simulink model "eovsa_corr_300mhz"  (R2012b)
(part 2 of 65)

      | % elseif strcmp(mode, 'fields of arbitrary size')
      | %     current_names = textscan(strtrim(strrep(strrep(get_param(blk, 'names'), ']', ''), '[', '')), '%s');
      | %     current_names = current_names{1};
      | %     numios = length(current_names);
      | %     if length(current_bins) ~= numios,
      | %         error('%d field names specified, but %d binary pts?', numios, length(current_bins));
      | %     end
      | % end
  vector_acc : Subsystem  mask{fpga_clk=300, fft_size=12, n_pps=50}
      mask prompts: fpga_clk "FPGA Clock Frequency (MHz)"; fft_size "FFT channels (2 ^ ?)"; n_pps "Accumulatioms per second"
  x_dv_count0 : Subsystem  Tag=xps:sw_reg  AncestorBlock=xps_library/software_register  mask(swreg){mode=one value, io_dir=To Processor, io_delay=0, sample_period=1, names=reg, bitwidths=32, arith_types=0, bin_pts=0, sim_port=on, show_format=off}
      mask prompts: io_dir "I/O direction"; io_delay "I/O delay"; sample_period "Sample period"; names "Name:"; bitwidths "Bitwidth:"; arith_types "Type (ufix=0, fix=1, bool=2):"; bin_pts "Binary pt:"; sim_port "Provide sim input/output?"; show_format "Print format string?"
      mask init:
      | swreg_init(gcb)
      settings: AttributesFormatString=1output
      mask TypeOptions mode: one value | fields of equal size | fields of arbitrary size
      mask Callback mode: swreg_cb(gcb);
      mask TypeOptions io_dir: To Processor | From Processor
      mask Callback io_dir:
      | mask_enables = get_param(gcb, 'MaskEnables');
      | mask_names = get_param(gcb, 'MaskNames');
      | if strcmp(get_param(gcb, 'io_dir'), 'To Processor'),
      |     mask_enables{ismember(mask_names, 'sample_period')} = 'off';
      | else
      |     mask_enables{ismember(mask_names, 'sample_period')} = 'on';
      | end
      | set_param(gcb, 'MaskEnables', mask_enables);
      mask Callback bitwidths:
      | swreg_maskcheck(gcb);
      | % blk = gcb;
      | % mode = get_param(blk, 'mode');
      | % current_widths = eval(get_param(blk, 'bitwidths'));
      | % if (strcmp(mode, 'one value') || strcmp(mode, 'fields of equal size')) && (length(current_widths) > 1),
      | %     error('Only one width may be specified for this mode.');
      | % elseif strcmp(mode, 'fields of arbitrary size')
      | %     current_names = textscan(strtrim(strrep(strrep(get_param(blk, 'names'), ']', ''), '[', '')), '%s');
      | %     current_names = current_names{1};
      | %     numios = length(current_names);
      | %     if length(current_widths) ~= numios,
      | %         error('%d field names specified, but %d widths?', numios, length(current_widths));
      | %     end
      | % end
      | % total_width = 0;
      | % for ctr = 1 : length(current_widths),
      | %     total_width = total_width + current_widths(ctr);
      | % end
      | % if total_width > 32,
      | %     error('Total width must be 32 or less, set to %d.', total_width);
      | % end
      mask Callback arith_types:
      | [numios, ~, ~, ~, current_types] = swreg_maskcheck(gcb);
      | % blk = gcb;
      | % mode = get_param(blk, 'mode');
      | % current_types = eval(get_param(blk, 'arith_types'));
      | % numios = length(current_types);
      | % if (strcmp(mode, 'one value') || strcmp(mode, 'fields of equal size')) && (length(current_types) > 1),
      | %     error('Only one type may be specified for this mode.');
      | % elseif strcmp(mode, 'fields of arbitrary size')
      | %     current_names = textscan(strtrim(strrep(strrep(get_param(blk, 'names'), ']', ''), '[', '')), '%s');
      | %     current_names = current_names{1};
      | %     numios = length(current_names);
      | %     if length(current_types) ~= numios,
      | %         error('%d field names specified, but %d types?', numios, length(current_types));
      | %     end
      | % end
      | problem = 0;
      | for ctr = 1 : numios,
      |     t = current_types(ctr);
      |     if (t < 0) || (t > 2),
      |         problem = t;
      |         ctr = numios + 1;
      |     end
      | end
      | if problem ~= 0,
      |     error('Type cannot be %i, must be 0, 1 or 2.', problem);
      | end
      mask Callback bin_pts:
      | swreg_maskcheck(gcb);
      | % blk = gcb;
      | % mode = get_param(blk, 'mode');
      | % current_bins = eval(get_param(blk, 'bin_pts'));
      | % if (strcmp(mode, 'one value') || strcmp(mode, 'fields of equal size')) && (length(current_bins) > 1),
      | %     error('Only one binary pt may be specified for this mode.');
      | % elseif strcmp(mode, 'fields of arbitrary size')
      | %     current_names = textscan(strtrim(strrep(strrep(get_param(blk, 'names'), ']', ''), '[', '')), '%s');
      | %     current_names = current_names{1};
      | %     numios = length(current_names);
      | %     if length(current_bins) ~= numios,
      | %         error('%d field names specified, but %d binary pts?', numios, length(current_bins));
      | %     end
      | % end
  x_dv_count1 : Subsystem  Tag=xps:sw_reg  AncestorBlock=xps_library/software_register  mask(swreg){mode=one value, io_dir=To Processor, io_delay=0, sample_period=1, names=reg, bitwidths=32, arith_types=0, bin_pts=0, sim_port=on, show_format=off}
      mask prompts: io_dir "I/O direction"; io_delay "I/O delay"; sample_period "Sample period"; names "Name:"; bitwidths "Bitwidth:"; arith_types "Type (ufix=0, fix=1, bool=2):"; bin_pts "Binary pt:"; sim_port "Provide sim input/output?"; show_format "Print format string?"
      mask init:
      | swreg_init(gcb)
      settings: AttributesFormatString=1output
      mask TypeOptions mode: one value | fields of equal size | fields of arbitrary size
      mask Callback mode: swreg_cb(gcb);
      mask TypeOptions io_dir: To Processor | From Processor
      mask Callback io_dir:
      | mask_enables = get_param(gcb, 'MaskEnables');
      | mask_names = get_param(gcb, 'MaskNames');
      | if strcmp(get_param(gcb, 'io_dir'), 'To Processor'),
      |     mask_enables{ismember(mask_names, 'sample_period')} = 'off';
      | else
      |     mask_enables{ismember(mask_names, 'sample_period')} = 'on';
      | end
      | set_param(gcb, 'MaskEnables', mask_enables);
      mask Callback bitwidths:
      | swreg_maskcheck(gcb);
      | % blk = gcb;
      | % mode = get_param(blk, 'mode');
      | % current_widths = eval(get_param(blk, 'bitwidths'));
      | % if (strcmp(mode, 'one value') || strcmp(mode, 'fields of equal size')) && (length(current_widths) > 1),
      | %     error('Only one width may be specified for this mode.');
      | % elseif strcmp(mode, 'fields of arbitrary size')
      | %     current_names = textscan(strtrim(strrep(strrep(get_param(blk, 'names'), ']', ''), '[', '')), '%s');
      | %     current_names = current_names{1};
      | %     numios = length(current_names);
      | %     if length(current_widths) ~= numios,
      | %         error('%d field names specified, but %d widths?', numios, length(current_widths));
      | %     end
      | % end
      | % total_width = 0;
      | % for ctr = 1 : length(current_widths),
      | %     total_width = total_width + current_widths(ctr);
      | % end
      | % if total_width > 32,
      | %     error('Total width must be 32 or less, set to %d.', total_width);
      | % end
      mask Callback arith_types:
      | [numios, ~, ~, ~, current_types] = swreg_maskcheck(gcb);
      | % blk = gcb;
      | % mode = get_param(blk, 'mode');
      | % current_types = eval(get_param(blk, 'arith_types'));
      | % numios = length(current_types);
      | % if (strcmp(mode, 'one value') || strcmp(mode, 'fields of equal size')) && (length(current_types) > 1),
      | %     error('Only one type may be specified for this mode.');
      | % elseif strcmp(mode, 'fields of arbitrary size')
      | %     current_names = textscan(strtrim(strrep(strrep(get_param(blk, 'names'), ']', ''), '[', '')), '%s');
      | %     current_names = current_names{1};
      | %     numios = length(current_names);
      | %     if length(current_types) ~= numios,
      | %         error('%d field names specified, but %d types?', numios, length(current_types));
      | %     end
      | % end
      | problem = 0;
      | for ctr = 1 : numios,
      |     t = current_types(ctr);
      |     if (t < 0) || (t > 2),
      |         problem = t;
      |         ctr = numios + 1;
      |     end
      | end
      | if problem ~= 0,
      |     error('Type cannot be %i, must be 0, 1 or 2.', problem);
      | end
      mask Callback bin_pts:
      | swreg_maskcheck(gcb);
      | % blk = gcb;
      | % mode = get_param(blk, 'mode');
      | % current_bins = eval(get_param(blk, 'bin_pts'));
      | % if (strcmp(mode, 'one value') || strcmp(mode, 'fields of equal size')) && (length(current_bins) > 1),
      | %     error('Only one binary pt may be specified for this mode.');
      | % elseif strcmp(mode, 'fields of arbitrary size')
      | %     current_names = textscan(strtrim(strrep(strrep(get_param(blk, 'names'), ']', ''), '[', '')), '%s');
      | %     current_names = current_names{1};
      | %     numios = length(current_names);
      | %     if length(current_bins) ~= numios,
      | %         error('%d field names specified, but %d binary pts?', numios, length(current_bins));
      | %     end
      | % end
  x_in_sync_count : Subsystem  Tag=xps:sw_reg  AncestorBlock=xps_library/software_register  mask(swreg){mode=one value, io_dir=To Processor, io_delay=0, sample_period=1, names=reg, bitwidths=32, arith_types=0, bin_pts=0, sim_port=on, show_format=off}
      mask prompts: io_dir "I/O direction"; io_delay "I/O delay"; sample_period "Sample period"; names "Name:"; bitwidths "Bitwidth:"; arith_types "Type (ufix=0, fix=1, bool=2):"; bin_pts "Binary pt:"; sim_port "Provide sim input/output?"; show_format "Print format string?"
      mask init:
      | swreg_init(gcb)
      settings: AttributesFormatString=1output
      mask TypeOptions mode: one value | fields of equal size | fields of arbitrary size
      mask Callback mode: swreg_cb(gcb);
      mask TypeOptions io_dir: To Processor | From Processor
      mask Callback io_dir:
      | mask_enables = get_param(gcb, 'MaskEnables');
      | mask_names = get_param(gcb, 'MaskNames');
      | if strcmp(get_param(gcb, 'io_dir'), 'To Processor'),
      |     mask_enables{ismember(mask_names, 'sample_period')} = 'off';
      | else
      |     mask_enables{ismember(mask_names, 'sample_period')} = 'on';
      | end
      | set_param(gcb, 'MaskEnables', mask_enables);
      mask Callback bitwidths:
      | swreg_maskcheck(gcb);
      | % blk = gcb;
      | % mode = get_param(blk, 'mode');
      | % current_widths = eval(get_param(blk, 'bitwidths'));
      | % if (strcmp(mode, 'one value') || strcmp(mode, 'fields of equal size')) && (length(current_widths) > 1),
      | %     error('Only one width may be specified for this mode.');
      | % elseif strcmp(mode, 'fields of arbitrary size')
      | %     current_names = textscan(strtrim(strrep(strrep(get_param(blk, 'names'), ']', ''), '[', '')), '%s');
      | %     current_names = current_names{1};
      | %     numios = length(current_names);
      | %     if length(current_widths) ~= numios,
      | %         error('%d field names specified, but %d widths?', numios, length(current_widths));
      | %     end
      | % end
      | % total_width = 0;
      | % for ctr = 1 : length(current_widths),
      | %     total_width = total_width + current_widths(ctr);
      | % end
      | % if total_width > 32,
      | %     error('Total width must be 32 or less, set to %d.', total_width);
      | % end
      mask Callback arith_types:
      | [numios, ~, ~, ~, current_types] = swreg_maskcheck(gcb);
      | % blk = gcb;
      | % mode = get_param(blk, 'mode');
      | % current_types = eval(get_param(blk, 'arith_types'));
      | % numios = length(current_types);
      | % if (strcmp(mode, 'one value') || strcmp(mode, 'fields of equal size')) && (length(current_types) > 1),
      | %     error('Only one type may be specified for this mode.');
      | % elseif strcmp(mode, 'fields of arbitrary size')
      | %     current_names = textscan(strtrim(strrep(strrep(get_param(blk, 'names'), ']', ''), '[', '')), '%s');
      | %     current_names = current_names{1};
      | %     numios = length(current_names);
      | %     if length(current_types) ~= numios,
      | %         error('%d field names specified, but %d types?', numios, length(current_types));
      | %     end
      | % end
      | problem = 0;
      | for ctr = 1 : numios,
      |     t = current_types(ctr);
      |     if (t < 0) || (t > 2),
      |         problem = t;
      |         ctr = numios + 1;
      |     end
      | end
      | if problem ~= 0,
      |     error('Type cannot be %i, must be 0, 1 or 2.', problem);
      | end
      mask Callback bin_pts:
      | swreg_maskcheck(gcb);
      | % blk = gcb;
      | % mode = get_param(blk, 'mode');
      | % current_bins = eval(get_param(blk, 'bin_pts'));
      | % if (strcmp(mode, 'one value') || strcmp(mode, 'fields of equal size')) && (length(current_bins) > 1),
      | %     error('Only one binary pt may be specified for this mode.');
      | % elseif strcmp(mode, 'fields of arbitrary size')
      | %     current_names = textscan(strtrim(strrep(strrep(get_param(blk, 'names'), ']', ''), '[', '')), '%s');
      | %     current_names = current_names{1};
      | %     numios = length(current_names);
      | %     if length(current_bins) ~= numios,
      | %         error('%d field names specified, but %d binary pts?', numios, length(current_bins));
      | %     end
      | % end
  x_out_count : Subsystem  Tag=xps:sw_reg  AncestorBlock=xps_library/software_register  mask(swreg){mode=one value, io_dir=To Processor, io_delay=0, sample_period=1, names=reg, bitwidths=32, arith_types=0, bin_pts=0, sim_port=on, show_format=off}
      mask prompts: io_dir "I/O direction"; io_delay "I/O delay"; sample_period "Sample period"; names "Name:"; bitwidths "Bitwidth:"; arith_types "Type (ufix=0, fix=1, bool=2):"; bin_pts "Binary pt:"; sim_port "Provide sim input/output?"; show_format "Print format string?"
      mask init:
      | swreg_init(gcb)
      settings: AttributesFormatString=1output
      mask TypeOptions mode: one value | fields of equal size | fields of arbitrary size
      mask Callback mode: swreg_cb(gcb);
      mask TypeOptions io_dir: To Processor | From Processor
      mask Callback io_dir:
      | mask_enables = get_param(gcb, 'MaskEnables');
      | mask_names = get_param(gcb, 'MaskNames');
      | if strcmp(get_param(gcb, 'io_dir'), 'To Processor'),
      |     mask_enables{ismember(mask_names, 'sample_period')} = 'off';
      | else
      |     mask_enables{ismember(mask_names, 'sample_period')} = 'on';
      | end
      | set_param(gcb, 'MaskEnables', mask_enables);
      mask Callback bitwidths:
      | swreg_maskcheck(gcb);
      | % blk = gcb;
      | % mode = get_param(blk, 'mode');
      | % current_widths = eval(get_param(blk, 'bitwidths'));
      | % if (strcmp(mode, 'one value') || strcmp(mode, 'fields of equal size')) && (length(current_widths) > 1),
      | %     error('Only one width may be specified for this mode.');
      | % elseif strcmp(mode, 'fields of arbitrary size')
      | %     current_names = textscan(strtrim(strrep(strrep(get_param(blk, 'names'), ']', ''), '[', '')), '%s');
      | %     current_names = current_names{1};
      | %     numios = length(current_names);
      | %     if length(current_widths) ~= numios,
      | %         error('%d field names specified, but %d widths?', numios, length(current_widths));
      | %     end
      | % end
      | % total_width = 0;
      | % for ctr = 1 : length(current_widths),
      | %     total_width = total_width + current_widths(ctr);
      | % end
      | % if total_width > 32,
      | %     error('Total width must be 32 or less, set to %d.', total_width);
      | % end
      mask Callback arith_types:
      | [numios, ~, ~, ~, current_types] = swreg_maskcheck(gcb);
      | % blk = gcb;
      | % mode = get_param(blk, 'mode');
      | % current_types = eval(get_param(blk, 'arith_types'));
      | % numios = length(current_types);
      | % if (strcmp(mode, 'one value') || strcmp(mode, 'fields of equal size')) && (length(current_types) > 1),
      | %     error('Only one type may be specified for this mode.');
      | % elseif strcmp(mode, 'fields of arbitrary size')
      | %     current_names = textscan(strtrim(strrep(strrep(get_param(blk, 'names'), ']', ''), '[', '')), '%s');
      | %     current_names = current_names{1};
      | %     numios = length(current_names);
      | %     if length(current_types) ~= numios,
      | %         error('%d field names specified, but %d types?', numios, length(current_types));
      | %     end
      | % end
      | problem = 0;
      | for ctr = 1 : numios,
      |     t = current_types(ctr);
      |     if (t < 0) || (t > 2),
      |         problem = t;
      |         ctr = numios + 1;
      |     end
      | end
      | if problem ~= 0,
      |     error('Type cannot be %i, must be 0, 1 or 2.', problem);
      | end
      mask Callback bin_pts:
      | swreg_maskcheck(gcb);
      | % blk = gcb;
      | % mode = get_param(blk, 'mode');
      | % current_bins = eval(get_param(blk, 'bin_pts'));
      | % if (strcmp(mode, 'one value') || strcmp(mode, 'fields of equal size')) && (length(current_bins) > 1),
      | %     error('Only one binary pt may be specified for this mode.');
      | % elseif strcmp(mode, 'fields of arbitrary size')
      | %     current_names = textscan(strtrim(strrep(strrep(get_param(blk, 'names'), ']', ''), '[', '')), '%s');
      | %     current_names = current_names{1};
      | %     numios = length(current_names);
      | %     if length(current_bins) ~= numios,
      | %         error('%d field names specified, but %d binary pts?', numios, length(current_bins));
      | %     end
      | % end
  x_packet_count : Subsystem  Tag=xps:sw_reg  AncestorBlock=xps_library/software_register  mask(swreg){mode=one value, io_dir=To Processor, io_delay=0, sample_period=1, names=reg, bitwidths=32, arith_types=0, bin_pts=0, sim_port=on, show_format=off}
      mask prompts: io_dir "I/O direction"; io_delay "I/O delay"; sample_period "Sample period"; names "Name:"; bitwidths "Bitwidth:"; arith_types "Type (ufix=0, fix=1, bool=2):"; bin_pts "Binary pt:"; sim_port "Provide sim input/output?"; show_format "Print format string?"
      mask init:
      | swreg_init(gcb)
      settings: AttributesFormatString=1output
      mask TypeOptions mode: one value | fields of equal size | fields of arbitrary size
      mask Callback mode: swreg_cb(gcb);
      mask TypeOptions io_dir: To Processor | From Processor
      mask Callback io_dir:
      | mask_enables = get_param(gcb, 'MaskEnables');
      | mask_names = get_param(gcb, 'MaskNames');
      | if strcmp(get_param(gcb, 'io_dir'), 'To Processor'),
      |     mask_enables{ismember(mask_names, 'sample_period')} = 'off';
      | else
      |     mask_enables{ismember(mask_names, 'sample_period')} = 'on';
      | end
      | set_param(gcb, 'MaskEnables', mask_enables);
      mask Callback bitwidths:
      | swreg_maskcheck(gcb);
      | % blk = gcb;
      | % mode = get_param(blk, 'mode');
      | % current_widths = eval(get_param(blk, 'bitwidths'));
      | % if (strcmp(mode, 'one value') || strcmp(mode, 'fields of equal size')) && (length(current_widths) > 1),
      | %     error('Only one width may be specified for this mode.');
      | % elseif strcmp(mode, 'fields of arbitrary size')
      | %     current_names = textscan(strtrim(strrep(strrep(get_param(blk, 'names'), ']', ''), '[', '')), '%s');
      | %     current_names = current_names{1};
      | %     numios = length(current_names);
      | %     if length(current_widths) ~= numios,
      | %         error('%d field names specified, but %d widths?', numios, length(current_widths));
      | %     end
      | % end
      | % total_width = 0;
      | % for ctr = 1 : length(current_widths),
      | %     total_width = total_width + current_widths(ctr);
      | % end
      | % if total_width > 32,
      | %     error('Total width must be 32 or less, set to %d.', total_width);
      | % end
      mask Callback arith_types:
      | [numios, ~, ~, ~, current_types] = swreg_maskcheck(gcb);
      | % blk = gcb;
      | % mode = get_param(blk, 'mode');
      | % current_types = eval(get_param(blk, 'arith_types'));
      | % numios = length(current_types);
      | % if (strcmp(mode, 'one value') || strcmp(mode, 'fields of equal size')) && (length(current_types) > 1),
      | %     error('Only one type may be specified for this mode.');
      | % elseif strcmp(mode, 'fields of arbitrary size')
      | %     current_names = textscan(strtrim(strrep(strrep(get_param(blk, 'names'), ']', ''), '[', '')), '%s');
      | %     current_names = current_names{1};
      | %     numios = length(current_names);
      | %     if length(current_types) ~= numios,
      | %         error('%d field names specified, but %d types?', numios, length(current_types));
      | %     end
      | % end
      | problem = 0;
      | for ctr = 1 : numios,
      |     t = current_types(ctr);
      |     if (t < 0) || (t > 2),
      |         problem = t;
      |         ctr = numios + 1;
      |     end
      | end
      | if problem ~= 0,
      |     error('Type cannot be %i, must be 0, 1 or 2.', problem);
      | end
      mask Callback bin_pts:
      | swreg_maskcheck(gcb);
      | % blk = gcb;
      | % mode = get_param(blk, 'mode');
      | % current_bins = eval(get_param(blk, 'bin_pts'));
      | % if (strcmp(mode, 'one value') || strcmp(mode, 'fields of equal size')) && (length(current_bins) > 1),
      | %     error('Only one binary pt may be specified for this mode.');
      | % elseif strcmp(mode, 'fields of arbitrary size')
      | %     current_names = textscan(strtrim(strrep(strrep(get_param(blk, 'names'), ']', ''), '[', '')), '%s');
      | %     current_names = current_names{1};
      | %     numios = length(current_names);
      | %     if length(current_bins) ~= numios,
      | %         error('%d field names specified, but %d binary pts?', numios, length(current_bins));
      | %     end
      | % end
  x_packet_err0 : Subsystem  Tag=xps:sw_reg  AncestorBlock=xps_library/software_register  mask(swreg){mode=one value, io_dir=To Processor, io_delay=0, sample_period=1, names=reg, bitwidths=32, arith_types=0, bin_pts=0, sim_port=on, show_format=off}
      mask prompts: io_dir "I/O direction"; io_delay "I/O delay"; sample_period "Sample period"; names "Name:"; bitwidths "Bitwidth:"; arith_types "Type (ufix=0, fix=1, bool=2):"; bin_pts "Binary pt:"; sim_port "Provide sim input/output?"; show_format "Print format string?"
      mask init:
      | swreg_init(gcb)
      settings: AttributesFormatString=1output
      mask TypeOptions mode: one value | fields of equal size | fields of arbitrary size
      mask Callback mode: swreg_cb(gcb);
      mask TypeOptions io_dir: To Processor | From Processor
      mask Callback io_dir:
      | mask_enables = get_param(gcb, 'MaskEnables');
      | mask_names = get_param(gcb, 'MaskNames');
      | if strcmp(get_param(gcb, 'io_dir'), 'To Processor'),
      |     mask_enables{ismember(mask_names, 'sample_period')} = 'off';
      | else
      |     mask_enables{ismember(mask_names, 'sample_period')} = 'on';
      | end
      | set_param(gcb, 'MaskEnables', mask_enables);
      mask Callback bitwidths:
      | swreg_maskcheck(gcb);
      | % blk = gcb;
      | % mode = get_param(blk, 'mode');
      | % current_widths = eval(get_param(blk, 'bitwidths'));
      | % if (strcmp(mode, 'one value') || strcmp(mode, 'fields of equal size')) && (length(current_widths) > 1),
      | %     error('Only one width may be specified for this mode.');
      | % elseif strcmp(mode, 'fields of arbitrary size')
      | %     current_names = textscan(strtrim(strrep(strrep(get_param(blk, 'names'), ']', ''), '[', '')), '%s');
      | %     current_names = current_names{1};
      | %     numios = length(current_names);
      | %     if length(current_widths) ~= numios,
      | %         error('%d field names specified, but %d widths?', numios, length(current_widths));
      | %     end
      | % end
      | % total_width = 0;
      | % for ctr = 1 : length(current_widths),
      | %     total_width = total_width + current_widths(ctr);
      | % end
      | % if total_width > 32,
      | %     error('Total width must be 32 or less, set to %d.', total_width);
      | % end
      mask Callback arith_types:
      | [numios, ~, ~, ~, current_types] = swreg_maskcheck(gcb);
      | % blk = gcb;
      | % mode = get_param(blk, 'mode');
      | % current_types = eval(get_param(blk, 'arith_types'));
      | % numios = length(current_types);
      | % if (strcmp(mode, 'one value') || strcmp(mode, 'fields of equal size')) && (length(current_types) > 1),
      | %     error('Only one type may be specified for this mode.');
      | % elseif strcmp(mode, 'fields of arbitrary size')
      | %     current_names = textscan(strtrim(strrep(strrep(get_param(blk, 'names'), ']', ''), '[', '')), '%s');
      | %     current_names = current_names{1};
      | %     numios = length(current_names);
      | %     if length(current_types) ~= numios,
      | %         error('%d field names specified, but %d types?', numios, length(current_types));
      | %     end
      | % end
      | problem = 0;
      | for ctr = 1 : numios,
      |     t = current_types(ctr);
      |     if (t < 0) || (t > 2),
      |         problem = t;
      |         ctr = numios + 1;
      |     end
      | end
      | if problem ~= 0,
      |     error('Type cannot be %i, must be 0, 1 or 2.', problem);
      | end
      mask Callback bin_pts:
      | swreg_maskcheck(gcb);
      | % blk = gcb;
      | % mode = get_param(blk, 'mode');
      | % current_bins = eval(get_param(blk, 'bin_pts'));
      | % if (strcmp(mode, 'one value') || strcmp(mode, 'fields of equal size')) && (length(current_bins) > 1),
      | %     error('Only one binary pt may be specified for this mode.');
      | % elseif strcmp(mode, 'fields of arbitrary size')
      | %     current_names = textscan(strtrim(strrep(strrep(get_param(blk, 'names'), ']', ''), '[', '')), '%s');
      | %     current_names = current_names{1};
      | %     numios = length(current_names);
      | %     if length(current_bins) ~= numios,
      | %         error('%d field names specified, but %d binary pts?', numios, length(current_bins));
      | %     end
      | % end
  x_packet_err1 : Subsystem  Tag=xps:sw_reg  AncestorBlock=xps_library/software_register  mask(swreg){mode=one value, io_dir=To Processor, io_delay=0, sample_period=1, names=reg, bitwidths=32, arith_types=0, bin_pts=0, sim_port=on, show_format=off}
      mask prompts: io_dir "I/O direction"; io_delay "I/O delay"; sample_period "Sample period"; names "Name:"; bitwidths "Bitwidth:"; arith_types "Type (ufix=0, fix=1, bool=2):"; bin_pts "Binary pt:"; sim_port "Provide sim input/output?"; show_format "Print format string?"
      mask init:
      | swreg_init(gcb)
      settings: AttributesFormatString=1output
      mask TypeOptions mode: one value | fields of equal size | fields of arbitrary size
      mask Callback mode: swreg_cb(gcb);
      mask TypeOptions io_dir: To Processor | From Processor
      mask Callback io_dir:
      | mask_enables = get_param(gcb, 'MaskEnables');
      | mask_names = get_param(gcb, 'MaskNames');
      | if strcmp(get_param(gcb, 'io_dir'), 'To Processor'),
      |     mask_enables{ismember(mask_names, 'sample_period')} = 'off';
      | else
      |     mask_enables{ismember(mask_names, 'sample_period')} = 'on';
      | end
      | set_param(gcb, 'MaskEnables', mask_enables);
      mask Callback bitwidths:
      | swreg_maskcheck(gcb);
      | % blk = gcb;
      | % mode = get_param(blk, 'mode');
      | % current_widths = eval(get_param(blk, 'bitwidths'));
      | % if (strcmp(mode, 'one value') || strcmp(mode, 'fields of equal size')) && (length(current_widths) > 1),
      | %     error('Only one width may be specified for this mode.');
      | % elseif strcmp(mode, 'fields of arbitrary size')
      | %     current_names = textscan(strtrim(strrep(strrep(get_param(blk, 'names'), ']', ''), '[', '')), '%s');
      | %     current_names = current_names{1};
      | %     numios = length(current_names);
      | %     if length(current_widths) ~= numios,
      | %         error('%d field names specified, but %d widths?', numios, length(current_widths));
      | %     end
      | % end
      | % total_width = 0;
      | % for ctr = 1 : length(current_widths),
      | %     total_width = total_width + current_widths(ctr);
      | % end
      | % if total_width > 32,
      | %     error('Total width must be 32 or less, set to %d.', total_width);
      | % end
      mask Callback arith_types:
      | [numios, ~, ~, ~, current_types] = swreg_maskcheck(gcb);
      | % blk = gcb;
      | % mode = get_param(blk, 'mode');
      | % current_types = eval(get_param(blk, 'arith_types'));
      | % numios = length(current_types);
      | % if (strcmp(mode, 'one value') || strcmp(mode, 'fields of equal size')) && (length(current_types) > 1),
      | %     error('Only one type may be specified for this mode.');
      | % elseif strcmp(mode, 'fields of arbitrary size')
      | %     current_names = textscan(strtrim(strrep(strrep(get_param(blk, 'names'), ']', ''), '[', '')), '%s');
      | %     current_names = current_names{1};
      | %     numios = length(current_names);
      | %     if length(current_types) ~= numios,
      | %         error('%d field names specified, but %d types?', numios, length(current_types));
      | %     end
      | % end
      | problem = 0;
      | for ctr = 1 : numios,
      |     t = current_types(ctr);
      |     if (t < 0) || (t > 2),
      |         problem = t;
      |         ctr = numios + 1;
      |     end
      | end
      | if problem ~= 0,
      |     error('Type cannot be %i, must be 0, 1 or 2.', problem);
      | end
      mask Callback bin_pts:
      | swreg_maskcheck(gcb);
      | % blk = gcb;
      | % mode = get_param(blk, 'mode');
      | % current_bins = eval(get_param(blk, 'bin_pts'));
      | % if (strcmp(mode, 'one value') || strcmp(mode, 'fields of equal size')) && (length(current_bins) > 1),
      | %     error('Only one binary pt may be specified for this mode.');
      | % elseif strcmp(mode, 'fields of arbitrary size')
      | %     current_names = textscan(strtrim(strrep(strrep(get_param(blk, 'names'), ']', ''), '[', '')), '%s');
      | %     current_names = current_names{1};
      | %     numios = length(current_names);
      | %     if length(current_bins) ~= numios,
      | %         error('%d field names specified, but %d binary pts?', numios, length(current_bins));
      | %     end
      | % end
  xeng0_vacc : Subsystem
  xeng_hdl_uint : Subsystem  AncestorBlock=ox_lib/xeng/xeng_hdl_uint  mask(xeng){n_ants=16, n_bits=4, acc_len_bits=7, demux_factor=4, bram_latency=2, p_bits=2}
      mask prompts: n_ants "Number of antennas"; n_bits "Bit-width of samples in"; acc_len_bits "Accumulation length (2^?)"; bram_latency "BRAM latency"; p_bits "Number of parallel (dual-pol) samples? (2^?)"
      mask help: CASPER X engine with added internal valid data masking functionality, descramble and integral demux. Based on Aaron Parsons' and Lynn Urry's original X engine design.
      mask init:
      | xeng_core = [gcb, '/xeng_core'];
      | descramble = [gcb, '/xeng_descramble'];
      | %update description string
      | fmtstr = ['n_ants=', num2str(n_ants), ...
      |     '\nacc_len=', num2str(2^p_bits), 'x', num2str(2^acc_len_bits), ...
      |     '\ndemux=',num2str(demux_factor)];
      | set_param(gcb, 'AttributesFormatString', fmtstr);
      | 
      | %set xengine core parameters
      | set_param(xeng_core, 'n_ants', num2str(n_ants), ...
      |     'bitwidth', num2str(n_bits), ...
      |     'serial_acc_len_bits', num2str(acc_len_bits), ...
      |     'bram_latency', num2str(bram_latency), ...
      |     'p_factor_bits', num2str(p_bits));
      | 
      | %set descramble parameters
      | 
      | set_param(descramble, 'num_ants', num2str(n_ants), ...
      |     'demux_factor', demux_factor, ...
      |     'n_bits', num2str(n_bits), ...
      |     'acc_len', num2str(2^acc_len_bits), ...
      |     'p_acc_len', num2str(2^p_bits));
      settings: AttributesFormatString=n_ants=16\nacc_len=4x128\ndemux=4
      mask TypeOptions demux_factor: 1 | 2 | 4 | 8
  wires:
  [adc0_p0] -> Concat8/1
  [adc0_p1] -> Concat8/2
  [adc1_p0] -> Concat8/3
  [adc1_p1] -> Concat8/4
  bus_expand7/1(msb_out4) -> [data_adc0_p0]
  bus_expand7/2(out3) -> [data_adc0_p1]
  bus_expand7/3(out2) -> [data_adc1_p0]
  bus_expand7/4(lsb_out1) -> [data_adc1_p1]
  [adc0_en0] -> Logical8/2
  [adc0_p0] -> decat2/1(i1)
  decat2/1(o1) -> auto_shutoff0/1(In1)
  decat2/2(o2) -> auto_shutoff0/2(In2)
  decat2/3(o3) -> auto_shutoff0/3(In3)
  decat2/4(o4) -> auto_shutoff0/4(In4)
  [clr_status] -> auto_shutoff0/5(rst)
  [adc0_p1] -> decat1/1(i1)
  decat1/1(o1) -> auto_shutoff1/1(In1)
  decat1/2(o2) -> auto_shutoff1/2(In2)
  decat1/3(o3) -> auto_shutoff1/3(In3)
  decat1/4(o4) -> auto_shutoff1/4(In4)
  [clr_status] -> auto_shutoff1/5(rst)
  [adc1_p0] -> decat4/1(i1)
  decat4/1(o1) -> auto_shutoff2/1(In1)
  decat4/2(o2) -> auto_shutoff2/2(In2)
  decat4/3(o3) -> auto_shutoff2/3(In3)
  decat4/4(o4) -> auto_shutoff2/4(In4)
  [clr_status] -> auto_shutoff2/5(rst)
  [adc1_p1] -> decat3/1(i1)
  decat3/1(o1) -> auto_shutoff3/1(In1)
  decat3/2(o2) -> auto_shutoff3/2(In2)
  decat3/3(o3) -> auto_shutoff3/3(In3)
  decat3/4(o4) -> auto_shutoff3/4(In4)
  [clr_status] -> auto_shutoff3/5(rst)
  auto_shutoff1/1(en) -> Register7/3, Register7/1
  auto_shutoff0/1(en) -> Register6/3, Register6/1
  auto_shutoff2/1(en) -> Register8/3, Register8/1
  auto_shutoff3/1(en) -> Register10/3, Register10/1
  [clr_adc_bad] -> Register6/2, Register7/2, Register10/2, Register8/2
  Logical8/1 -> [status_adc0_en0]
  [adc0_en1] -> Logical6/2
  Logical6/1 -> [status_adc0_en1]
  [adc1_en0] -> Logical9/2
  Logical9/1 -> [status_adc1_en0]
  [adc1_en1] -> Logical10/2
  Logical10/1 -> [status_adc1_en1]
  timing/1(sync) -> [sync]
  edge_detect1/1(out) -> Mux/2
  FPGA_pps/1(pps) -> Delay4/1
  Mux/1 -> [pps]
  Convert/1 -> Mux/1
  timing/3(pps) -> [timing_pps]
  timing/4(armed) -> [armed]
  timing/5(synced) -> [synced]
  timing/6(adc_overflow) -> [adc_overflow_pulse]
  [fpga_pps] -> Convert/1
  [adc_sync] -> edge_detect1/1(in)
  [arm] -> timing/1(arm)
  [pps] -> timing/2(pps_in)
  Concat8/1 -> timing/3(data_in)
  [adc0_overflow] -> timing/4(adc0_over)
  [adc1_overflow] -> timing/5(adc1_over)
  timing/2(data_out) -> bus_expand7/1(bus_in)
  Register6/1 -> Inverter1/1
  Register7/1 -> Inverter2/1
  Register8/1 -> Inverter9/1
  Register10/1 -> Inverter10/1
  pkt_gate1/1(rst_o) -> Rx_Tx_FX0/1
  pkt_gate1/2(data_o) -> Rx_Tx_FX0/2
  pkt_gate1/3(dv_o) -> Rx_Tx_FX0/3, Delay61/1
  pkt_gate1/5(port_o) -> Rx_Tx_FX0/5
  pkt_gate1/6(eof_o) -> Delay64/1, Rx_Tx_FX0/6
  [dest_roach_FX1] -> Convert5/1
  [rst_ten_gbe] -> pkt_gate2/1(rst_i)
  pkt_gate2/1(rst_o) -> Rx_Tx_FX1/1
  pkt_gate2/2(data_o) -> Rx_Tx_FX1/2
  pkt_gate2/3(dv_o) -> Delay67/1, Rx_Tx_FX1/3
  pkt_gate2/6(eof_o) -> Delay68/1, Rx_Tx_FX1/6
  [ip0_f_tx_data] -> pkt_gate1/2(data_i)
  [ip1_f_tx_data] -> pkt_gate2/2(data_i)
  [ip0_f_tx_eof] -> pkt_gate1/6(eof_i)
  [ip1_f_tx_eof] -> pkt_gate2/6(eof_i)
  [dest_roach_FX0] -> Convert6/1
  pkt_gate1/4(ip_o) -> Rx_Tx_FX0/4
  [fx_udp_port] -> pkt_gate1/5(port_i)
  pkt_gate2/4(ip_o) -> Rx_Tx_FX1/4
  [fx_udp_port] -> pkt_gate2/5(port_i)
  Rx_Tx_FX0/1 -> Delay401/1
  Rx_Tx_FX0/2 -> Delay402/1
  Rx_Tx_FX0/3 -> Delay403/1
  Rx_Tx_FX0/6 -> Delay406/1
  Rx_Tx_FX0/7 -> Delay407/1
  Rx_Tx_FX0/9 -> Delay409/1
  Rx_Tx_FX0/10 -> Delay410/1
  Rx_Tx_FX0/11 -> Delay411/1
  Rx_Tx_FX1/1 -> Delay413/1
  Rx_Tx_FX1/2 -> Delay414/1
  Rx_Tx_FX1/3 -> Delay415/1
  Rx_Tx_FX1/6 -> Delay418/1
  Rx_Tx_FX1/7 -> Delay419/1
  Rx_Tx_FX1/9 -> Delay421/1
  Rx_Tx_FX1/10 -> Delay422/1
  Rx_Tx_FX1/11 -> Delay423/1
  Convert6/1 -> ip1/1(addr)
  f_x/1(data_out0) -> [ip0_f_tx_data]
  f_x/2(data_valid0) -> [ip0_f_tx_valid]
  f_x/3(dest_roach) -> [dest_roach_FX0]
  f_x/4(eof) -> [ip0_f_tx_eof]
  f_x/5(data_out1) -> [ip1_f_tx_data]
  f_x/6(data_valid1) -> [ip1_f_tx_valid]
  f_x/7(dest_roach1) -> [dest_roach_FX1]
  f_x/8(eof1) -> [ip1_f_tx_eof]
  f_x/9(x_packet_err0) -> [x_packet_err0]
  f_x/10(x_packet_err1) -> [x_packet_err1]
  tx_packet_count_fx0/1(sim_out) -> Terminator46/1
  tx_packet_count_fx1/1(sim_out) -> Terminator47/1
  tx_overflow_fx0/1(sim_out) -> Terminator49/1
  Counter15/1 -> tx_overflow_fx0/1(out_reg)
  Rx_Tx_FX0/5 -> Delay405/1
  tx_overflow_fx1/1(sim_out) -> Terminator68/1
  Counter17/1 -> tx_overflow_fx1/1(out_reg)
  Rx_Tx_FX1/5 -> Delay417/1
  Rx_Tx_FX1/12 -> Terminator69/1
  rx_packet_count_fx0/1(sim_out) -> Terminator70/1
  [gbe_rxvld0] -> Counter9/1
  rx_packet_count_fx1/1(sim_out) -> Terminator72/1
  Counter6/1 -> Slice13/1
  Counter7/1 -> Slice12/1
  Counter9/1 -> Slice14/1
  x_packet_err0/1(sim_out) -> Terminator39/1
  Counter30/1 -> x_packet_err0/1(out_reg)
  x_packet_err1/1(sim_out) -> Terminator43/1
  Counter31/1 -> x_packet_err1/1(out_reg)
  [x_packet_err0] -> Counter30/1
  [x_packet_err1] -> Counter31/1
  [rst_ten_gbe] -> Delay62/1
  [gbe_rxdata0] -> Delay245/1
  Delay35/1 -> unpack0/1(rst)
  Delay36/1 -> unpack0/2(gbe_din0)
  Delay54/1 -> unpack0/3(gbe_valid0)
  unpack0/1(dout) -> [dp0]
  unpack0/2(dvalid) -> [valid0]
  unpack0/3(hdr) -> [hdr0]
  unpack0/4(hdr_valid) -> [hdr_valid0]
  unpack0/5(eof) -> [eof0]
  Delay63/1 -> unpack1/1(rst)
  Delay76/1 -> unpack1/2(gbe_din0)
  Delay78/1 -> unpack1/3(gbe_valid0)
  unpack1/1(dout) -> [dp1]
  unpack1/2(dvalid) -> [valid1]
  unpack1/3(hdr) -> [hdr1]
  unpack1/4(hdr_valid) -> [hdr_valid1]
  unpack1/5(eof) -> [eof1]
  Constant5/1 -> rx_hdr/3(trig)
  [dp1] -> packet_buffer1/1(din)
  [valid1] -> packet_buffer1/2(dvalid)
  [eof1] -> packet_buffer1/3(eof)
  [hdr1] -> packet_buffer1/4(hdr)
  [hdr_valid1] -> packet_buffer1/5(hdr_valid)
  packet_count_x/1(sim_out) -> Terminator77/1
  Counter37/1 -> Delay138/1
  led_up1/1 -> Terminator81/1
  led_tx1/1 -> Terminator92/1
  tx_x_overflow/1(sim_out) -> Terminator93/1
  Counter38/1 -> Delay59/1
  Constant17/1 -> Tx_X/8
  pkt_gate3/2(data_o) -> Tx_X/2
  pkt_gate3/3(dv_o) -> Logical18/1, Tx_X/3
  pkt_gate3/4(ip_o) -> Tx_X/4
  pkt_gate3/5(port_o) -> Tx_X/5
  pkt_gate3/6(eof_o) -> Logical18/2, Tx_X/6
  Constant18/1 -> Tx_X/7
  [dpp_ip] -> pkt_gate3/4(ip_i)
  [dpp_port] -> pkt_gate3/5(port_i)
  [rst_ten_gbe] -> pkt_gate3/1(rst_i)
  pkt_gate3/1(rst_o) -> Tx_X/1
  Tx_X/1 -> Delay400/1
  Tx_X/2 -> Terminator91/1
  Tx_X/3 -> Delay100/1
  Tx_X/5 -> Delay8/1
  Tx_X/6 -> Terminator82/1
  Tx_X/7 -> Terminator80/1
  Tx_X/8 -> Terminator84/1
  Tx_X/9 -> Terminator79/1
  Tx_X/10 -> Terminator86/1
  Tx_X/11 -> Terminator78/1
  Tx_X/12 -> Terminator85/1
  packetizer_x1/1(pack_data) -> Delay177/1
  packetizer_x1/2(data_valid) -> Delay178/1
  packetizer_x1/3(pack_eof) -> Delay179/1
  Delay177/1 -> pkt_gate3/2(data_i)
  Delay179/1 -> pkt_gate3/6(eof_i)
  x_packet_count/1(sim_out) -> Terminator94/1
  Counter35/1 -> x_packet_count/1(out_reg)
  edge_detect12/1(out) -> Counter35/1
  Delay236/1 -> edge_detect12/1(in)
  x_dv_count1/1(sim_out) -> Terminator55/1
  x_dv_count0/1(sim_out) -> Terminator96/1
  Counter40/1 -> Slice17/1
  x_out_count/1(sim_out) -> Terminator59/1
  Counter50/1 -> Slice16/1
  adc/1(adc0_0_0) -> phase_switching/4(adc0_0_0)
  adc/2(adc0_0_1) -> phase_switching/5(adc0_0_1)
  adc/3(adc0_0_2) -> phase_switching/6(adc0_0_2)
  adc/4(adc0_0_3) -> phase_switching/7(adc0_0_3)
  adc/5(adc0_1_0) -> phase_switching/8(adc0_1_0)
  adc/6(adc0_1_1) -> phase_switching/9(adc0_1_1)
  adc/7(adc0_1_2) -> phase_switching/10(adc0_1_2)
  adc/8(adc0_1_3) -> phase_switching/11(adc0_1_3)
  adc/9(adc0_sync) -> phase_switching/12(adc0_sync), phase_switching/1(walsh_start)
  adc/10(adc0_oflow) -> phase_switching/13(adc0_overflow)
  adc/11(adc1_0_0) -> phase_switching/14(adc1_0_0)
  adc/12(adc1_0_1) -> phase_switching/15(adc1_0_1)
  adc/13(adc1_0_2) -> phase_switching/16(adc1_0_2)
  adc/14(adc1_0_3) -> phase_switching/17(adc1_0_3)
  adc/15(adc1_1_0) -> phase_switching/18(adc1_1_0)
  adc/16(adc1_1_1) -> phase_switching/19(adc1_1_1)
  adc/17(adc1_1_2) -> phase_switching/20(adc1_1_2)
  adc/18(adc1_1_3) -> phase_switching/21(adc1_1_3)
  adc/19(adc1_sync) -> phase_switching/22(adc1_sync)
  adc/20(adc1_oflow) -> phase_switching/23(adc1_overflow)
  [adc0_atten0] -> adc/2(adc0_atten0)
  [status_adc0_en1] -> adc/3(adc0_en1)
  [adc0_atten1] -> adc/4(adc0_atten1)
  [status_adc1_en0] -> adc/5(adc1_en0)
  [adc1_atten0] -> adc/6(adc1_atten0)
  [status_adc1_en1] -> adc/7(adc1_en1)
  [adc1_atten1] -> adc/8(adc1_atten1)
  phase_switching/2(adc0_pol0) -> [adc0_p0]
  phase_switching/3(adc0_pol1) -> [adc0_p1]
  phase_switching/7(adc1_pol1) -> [adc1_p1]
  phase_switching/6(adc1_pol0) -> [adc1_p0]
  [status_adc0_en0] -> adc/1(adc0_en0)
  phase_switching/1(sync_out) -> [sync_adc_out]
  phase_switching/4(adc_sync) -> [adc_sync]
  phase_switching/5(adc0_overflow_out) -> [adc0_overflow]
  phase_switching/8(adc1_overflow_out) -> [adc1_overflow]
  [pps_in] -> phase_switching/24(pps_in)
  [adc_snap_sel] -> adc/9(adc_snap_sel)
  [rx_hdr_snap_sel] -> Mux7/1
  [hdr1] -> Mux7/3
  [hdr0] -> Mux7/2
  [rx_hdr_snap_sel] -> Mux8/1
  [hdr_valid0] -> Mux8/2
  [hdr_valid1] -> Mux8/3
  Mux7/1 -> rx_hdr/1(din)
  Mux8/1 -> rx_hdr/2(we)
  Constant6/1 -> tx_pkt/3(trig)
  [tx_pkt_snap_sel] -> Mux9/1
  [ip0_f_tx_data] -> Mux9/2
  [ip1_f_tx_data] -> Mux9/3
  [tx_pkt_snap_sel] -> Mux10/1
  [ip0_f_tx_valid] -> Mux10/2
  [ip1_f_tx_valid] -> Mux10/3
  Mux9/1 -> tx_pkt/1(din)
  Mux10/1 -> tx_pkt/2(we)
  swreg/1(adc0_atten0) -> [adc0_atten0]
  swreg/57(x_in_snap_select) -> [x_in_snap_sel]
  swreg/2(adc0_atten1) -> [adc0_atten1]
  swreg/3(adc1_atten0) -> [adc1_atten0]
  swreg/4(adc1_atten1) -> [adc1_atten1]
  swreg/5(adc0_en0) -> [adc0_en0]
  swreg/6(adc0_en1) -> [adc0_en1]
  swreg/7(adc1_en0) -> [adc1_en0]
  swreg/8(adc1_en1) -> [adc1_en1]
  swreg/9(phs_switch0) -> [phs_switch_ant0]
  swreg/10(phs_switch1) -> [phs_switch_ant1]
  swreg/11(delay00) -> [delay00]
  swreg/12(delay01) -> [delay01]
  swreg/13(delay10) -> [delay10]
  swreg/14(delay11) -> [delay11]
  swreg/15(packet_delay) -> [packet_delay]
  swreg/16(fft_shift_out) -> [fft_shift]
  swreg/17(calibration_bram_address) -> [bram_address]
  swreg/18(calibration_bram_load_data) -> [bram_write_en]
  swreg/19(calibration_data_x0) -> [bram_data_x0]
  swreg/20(calibration_data_x1) -> [bram_data_x1]
  swreg/21(calibration_data_y0) -> [bram_data_y0]
  swreg/22(calibration_data_y1) -> [bram_data_y1]
  swreg/23(acc_length) -> [acc_len]
  swreg/24(acc_start_skip) -> [acc_start_skip]
  swreg/25(board_id) -> [board_id]
  swreg/26(boards_connected) -> [boards_connected]
  swreg/27(rst_ten_gbe) -> [rst_ten_gbe]
  swreg/28(dpp_ip_address) -> [dpp_ip]
  swreg/29(dpp_port_num) -> [dpp_port]
  swreg/30(roach_udp_port) -> [fx_udp_port]
  swreg/31(pps_in) -> [pps_in]
  swreg/32(fpga_pps) -> [fpga_pps]
  swreg/33(polarization) -> [use_circular]
  swreg/35(f_x_tvg) -> [ct_tvg]
  swreg/36(x_eng_tvg) -> [xeng_tvg_sel]
  swreg/39(clr_adc_bad) -> [clr_adc_bad]
  swreg/43(sw_arm) -> [arm]
  swreg/45(reset) -> Subsystem/1(In1)
  swreg/46(x_acc_length) -> [acc_len_x]
  swreg/47(x_packet_delay) -> [x_packet_delay]
  swreg/48(x_board_id) -> [x_board_id]
  swreg/50(x_polarization) -> [x_use_circular]
  swreg/51(op_select_x1) -> [x_op_select]
  swreg/52(adc_snap_select) -> [adc_snap_sel]
  swreg/53(fft_snap_select) -> [fft_snap_sel]
  swreg/54(pol_snap_select) -> [pol_snap_sel]
  swreg/55(tx_pkt_snap_select) -> [tx_pkt_snap_sel]
  swreg/56(rx_hdr_snap_select) -> [rx_hdr_snap_sel]
  swreg/40(clr_status) -> [clr_status]
  swreg/34(adc_protection) -> [adc_protection]
  Mux13/1 -> Logical8/1
  Constant1/1 -> Mux13/2
  [adc_protection] -> Mux13/1, Mux16/1, Mux15/1, Mux14/1
  Inverter1/1 -> Mux13/3
  Mux14/1 -> Logical6/1
  Mux15/1 -> Logical9/1
  Mux16/1 -> Logical10/1
  Constant2/1 -> Mux14/2
  Constant3/1 -> Mux15/2
  Constant36/1 -> Mux16/2
  Inverter2/1 -> Mux14/3
  Inverter9/1 -> Mux15/3
  Inverter10/1 -> Mux16/3
  Delay8/1 -> Counter38/1
  Delay100/1 -> led_tx1/1
  Delay400/1 -> led_up1/1
  Delay401/1 -> [gbe_up0]
  Delay402/1 -> [gbe_rx0]
  Delay403/1 -> [gbe_tx0]
  Delay405/1 -> Counter15/1
  Delay406/1 -> [gbe_rxdata0]
  Delay407/1 -> [gbe_rxvld0]
  Delay409/1 -> [gbe_rxport0]
  Delay410/1 -> [gbe_rxeof0]
  Delay411/1 -> [gbe_rx_bad0]
  Delay413/1 -> [gbe_up1]
  Delay414/1 -> [gbe_rx1]
  Delay415/1 -> [gbe_tx1]
  Delay417/1 -> Counter17/1
  Delay418/1 -> [gbe_rxdata1]
  Delay419/1 -> [gbe_rxvld1]
  Delay421/1 -> [gbe_rxport1]
  Delay422/1 -> [gbe_rxeof1]
  Delay423/1 -> [gbe_rx_bad1]
  swreg/49(x_rst) -> [x_mrst]
  swreg/37(tvg_rst) -> [tvg_rst]
  swreg/38(tvg_en) -> [tvg_en]
  [gbe_rxvld0] -> Delay252/1
  [x_arm] -> Delay465/1, Delay465/2
  Logical5/1 -> Delay54/1
  Delay62/1 -> Delay35/1
  Delay245/1 -> Delay36/1
  Delay252/1 -> Logical5/1
  [rst_ten_gbe] -> Delay469/1
  [gbe_rxdata1] -> Delay466/1
  [gbe_rxvld1] -> Delay467/1
  Logical7/1 -> Delay78/1
  Delay469/1 -> Delay63/1
  Delay466/1 -> Delay76/1
  Delay467/1 -> Logical7/1
  swreg/44(x_arm) -> [x_arm]
  Delay465/1 -> Logical5/2
  [x_arm] -> Delay468/1, Delay468/2
  Delay468/1 -> Logical7/2
  [dp0] -> packet_buffer0/1(din)
  [valid0] -> packet_buffer0/2(dvalid)
  [eof0] -> packet_buffer0/3(eof)
  [hdr0] -> packet_buffer0/4(hdr)
  [hdr_valid0] -> packet_buffer0/5(hdr_valid)
  Delay92/1 -> FIFO2/1
  Delay93/1 -> FIFO2/2
  FIFO2/1 -> Convert1/1, Convert2/1
  FIFO2/2 -> Terminator25/1
  FIFO2/3 -> Terminator28/1
  [read_header_data] -> Delay9/1
  [mrst5] -> FIFO2/4
  [sync] -> acc_sync/1(sync)
  [acc_len] -> acc_sync/2(acc_len)
  [adc_overflow_pulse] -> acc_sync/4(adc_over)
  acc_sync/1(acc_end) -> Delay93/1
  acc_sync/2(adc_overflow) -> Delay92/1
  Convert1/1 -> [adc_overflow]
  adc_overflow/1(sim_out) -> Terminator10/1
  Convert2/1 -> adc_overflow/1(out_reg)
  [acc_start_skip] -> acc_sync/3(acc_start_skip)
  [fft_shift] -> Delay389/1
  [acc_len] -> Delay390/1
  FIFO/1 -> Delay40/1
  FIFO/2 -> Terminator16/1
  FIFO/3 -> Terminator18/1
  [read_header_data] -> Delay11/1
  FIFO3/1 -> Delay16/1
  FIFO3/2 -> Terminator40/1
  FIFO3/3 -> Terminator41/1
  [read_header_data] -> Delay7/1
  [delay00] -> Concat1/1
  [delay01] -> Concat1/2
  [delay10] -> Concat1/3
  [delay11] -> Concat1/4
  Concat1/1 -> Delay96/1
  [sync] -> pulse generator2/1(sync)
  pulse generator2/1(pulse) -> Delay95/1
  Delay95/1 -> FIFO3/2
  Delay96/1 -> FIFO3/1
  [mrst1] -> FIFO3/4
  Logical1/1 -> Delay46/1
  FIFO1/1 -> Delay41/1
  [read_header_data] -> Delay10/1
  clip_count/1 -> Delay15/1
  FIFO1/2 -> Terminator21/1
  FIFO1/3 -> Terminator22/1
  [sync_polarimetry_out] -> Delay12/1
  pulse generator1/1(pulse) -> Delay44/1
  [mrst2] -> FIFO1/4
  [acc_start_skip] -> Delay399/1
  [pol_snap_sel] -> Delay335/1
  Mux11/1 -> BitBasher1/1
  [sync_polarimetry_out] -> Delay327/1
  Constant21/1 -> pol_snap/2(we)
  pulse generator3/1(pulse) -> pol_snap/3(trig)
  Concat15/1 -> Delay55/1
  Delay327/1 -> pulse generator3/1(sync)
  [sync] -> Delay379/1
  [timing_pps] -> Delay380/1
  [delay00] -> Delay381/1
  [data_adc0_p0] -> Delay382/1
  [delay01] -> Delay383/1
  [data_adc0_p1] -> Delay384/1
  [delay10] -> Delay385/1
  [data_adc1_p0] -> Delay386/1
  [delay11] -> Delay387/1
  [data_adc1_p1] -> Delay388/1
  Delay379/1 -> coarse_delay/1(sync)
  Delay380/1 -> coarse_delay/2(new_acc)
  Delay381/1 -> coarse_delay/3(delay00)
  Delay382/1 -> coarse_delay/4(adc0_pol0)
  Delay383/1 -> coarse_delay/5(delay01)
  Delay384/1 -> coarse_delay/6(adc0_pol1)
  Delay385/1 -> coarse_delay/7(delay10)
  Delay386/1 -> coarse_delay/8(adc1_pol0)
  Delay387/1 -> coarse_delay/9(delay11)
  Delay388/1 -> coarse_delay/10(adc1_pol1)
  Delay389/1 -> pfb_fft/1(fft_shift)
  Delay390/1 -> pfb_fft/2(acc_len)
  Delay399/1 -> pfb_fft/8(acc_start_skip)
  [acc_len] -> Delay194/1
  Constant40/1 -> Tx_P/7
  Tx_P/2 -> Terminator8/1
  Tx_P/3 -> Delay426/1
  Tx_P/4 -> ?
  Tx_P/5 -> Delay428/1
  Tx_P/6 -> Terminator17/1
  Tx_P/7 -> Terminator37/1
  Tx_P/8 -> Terminator27/1
  Tx_P/9 -> Terminator36/1
  Tx_P/10 -> Terminator34/1
  Tx_P/11 -> Terminator35/1
  Tx_P/12 -> Terminator29/1
  Constant41/1 -> Tx_P/8
  [acc_len] -> Delay45/1
  [use_circular] -> Delay66/1
  [board_id] -> Delay83/1
  [adc_overflow] -> Delay84/1
  [fft_shift] -> Delay85/1
  Slice11/1 -> Delay89/1
  Slice10/1 -> Delay90/1
  Slice9/1 -> Delay97/1
  Slice8/1 -> Delay446/1
  [clip_count] -> Delay455/1
  Slice7/1 -> Delay447/1
  Slice5/1 -> Delay448/1
  Slice4/1 -> Delay449/1
  Slice3/1 -> Delay450/1
  Slice6/1 -> Delay451/1
  Slice/1 -> Delay452/1
  Slice2/1 -> Delay453/1
  Slice1/1 -> Delay454/1
  [adc_calibration_data] -> Slice6/1, Slice7/1, Slice5/1, Slice4/1, Slice3/1, Slice/1, Slice2/1, Slice1/1
  [mrst4] -> Delay192/1
  Delay456/1 -> Delay31/1
  Delay458/1 -> Delay43/1
  [delay_val] -> Slice11/1, Slice10/1, Slice9/1, Slice8/1
  packet_count_p/1(sim_out) -> Terminator4/1
  Counter/1 -> Delay135/1
  sync/1(sim_out) -> Terminator5/1
  Counter60/1 -> sync/1(out_reg)
  Tx_P/1 -> Delay425/1
  led_up/1 -> Terminator6/1
  led_tx/1 -> Terminator9/1
  tx_p_overflow/1(sim_out) -> Terminator103/1
  Counter61/1 -> Delay57/1
  [mrst3] -> Delay81/1
  vector_acc/4(acc_num) -> Terminator104/1
  vector_acc/5(acc_numpps) -> Terminator105/1
  [packet_delay] -> Delay65/1
  [acc_start_skip] -> Delay232/1
  Delay192/1 -> vector_acc/1(mrst)
  power_cal/1(sync_out) -> vector_acc/2(sync), Counter60/1
  Delay194/1 -> vector_acc/3(acc_length)
  Delay232/1 -> vector_acc/20(acc_start_skip)
  Delay425/1 -> led_up/1
  Delay426/1 -> led_tx/1
  Delay428/1 -> Counter61/1
  [phs_switch_ant0] -> phase_switching/2(phs_ant0)
  [phs_switch_ant1] -> phase_switching/3(phs_ant1)
  [input_rst] -> adc/10(rst)
  [input_sel] -> adc/11(ip_select)
  swreg/41(input_rst) -> [input_rst]
  swreg/42(input_select) -> [input_sel]
  vector_acc/1(data) -> Delay456/1
  vector_acc/2(data_valid) -> Delay458/1
  vector_acc/3(acc_start) -> [read_header_data]
  Logical11/1 -> Counter/1
  [ip0_f_tx_valid] -> pkt_gate1/3(dv_i)
  [rst_ten_gbe] -> pkt_gate1/1(rst_i)
  Logical14/1 -> Counter6/1
  [ip1_f_tx_valid] -> pkt_gate2/3(dv_i)
  Slice12/1 -> Delay75/1
  Delay75/1 -> tx_packet_count_fx1/1(out_reg)
  Logical16/1 -> Counter7/1
  Slice13/1 -> Delay132/1
  Delay132/1 -> tx_packet_count_fx0/1(out_reg)
  Delay135/1 -> packet_count_p/1(out_reg)
  Delay178/1 -> pkt_gate3/3(dv_i)
  Delay138/1 -> packet_count_x/1(out_reg)
  Logical18/1 -> Counter37/1
  pkt_gate/3(dv_o) -> Logical11/1, Tx_P/3
  pkt_gate/6(eof_o) -> Logical11/2, Tx_P/6
  [rst_ten_gbe] -> pkt_gate/1(rst_i)
  packetizer_P/1(pack_data) -> pkt_gate/2(data_i)
  [dpp_ip] -> pkt_gate/4(ip_i)
  [dpp_port] -> pkt_gate/5(port_i)
  packetizer_P/2(data_valid) -> pkt_gate/3(dv_i)
  packetizer_P/3(pack_eof) -> pkt_gate/6(eof_i)
  pkt_gate/1(rst_o) -> Tx_P/1
  pkt_gate/2(data_o) -> Tx_P/2
  pkt_gate/4(ip_o) -> Tx_P/4
  pkt_gate/5(port_o) -> Tx_P/5
  ip1/1(data_out) -> pkt_gate1/4(ip_i)
  pkt_gate2/5(port_o) -> Rx_Tx_FX1/5
  ip0/1(data_out) -> pkt_gate2/4(ip_i)
  [rd_addr] -> packet_buffer0/6(rd_addr_in)
  [rd_valid0] -> packet_buffer0/7(rd_valid_in)
  packet_buffer0/5(rd_addr_out) -> [rd_addr]
  packet_buffer0/6(rd_valid_out0) -> [rd_valid0]
  [rd_addr] -> packet_buffer1/6(rd_addr_in)
  [rd_valid1] -> packet_buffer1/7(rd_valid_in)
  [hdr0] -> Slice19/1
  [hdr_valid0] -> Delay26/1
  Slice19/1 -> Delay25/1
  Delay25/1 -> Delay24/1
  Delay26/1 -> Delay24/2
  [hdr1] -> Slice25/1
  [hdr_valid1] -> Delay48/1
  Slice25/1 -> Delay33/1
  Delay33/1 -> Delay27/1
  Delay48/1 -> Delay27/2
  Delay24/1 -> BitBasher/1
  Delay27/1 -> BitBasher/2
  rx_mcount_fx0/1(sim_out) -> Terminator3/1
  BitBasher/1 -> rx_mcount_fx0/1(out_reg)
  BitBasher/2 -> rx_mcounts/1(out_reg)
  rx_mcounts/1(sim_out) -> Terminator60/1
  rx_mcount_fx1/1(sim_out) -> Terminator106/1
  BitBasher/3 -> rx_mcount_fx1/1(out_reg)
  output_burst_len/1 -> xeng0_vacc/7(rb_burst_len_mi)
  [acc_len_x] -> xeng0_vacc/2(acc_len_mi)
  [x_mrst] -> xeng0_vacc/1(rst)
  vacc_target_mcnt/1(in_reg) -> pipeline21/1(d)
  armer/3(vld_out) -> xeng0_vacc/5(we)
  armer/1(sync_out) -> xeng0_vacc/3(sync_in)
  armer/4(mcnt_out) -> xeng0_vacc/6(pcnt_in)
  armer/2(data_out) -> xeng0_vacc/4(data_in)
  [all_x_dout] -> armer/6(data)
  [all_x_mcnt] -> armer/3(mcnt)
  [all_x_sync] -> armer/4(sync)
  [all_x_vld] -> armer/2(vld)
  [x_mrst] -> armer/5(rst)
  pipeline21/1(q) -> armer/1(target_mcnt)
  xeng0_vacc/1(new_acc) -> [vacc_new_acc]
  xeng0_vacc/2(data_out) -> Delay1/1
  xeng0_vacc/3(valid_out) -> Delay2/1
  xeng0_vacc/4(timestamp) -> Delay3/1
  Constant4/1 -> packetizer_x1/5(use_circular)
  [x_board_id] -> packetizer_x1/6(x_eng_id)
  [acc_len_x] -> packetizer_x1/4(acc_len)
  [vacc_vld] -> packetizer_x1/3(acc_valid), Delay236/1
  [vacc_dout] -> packetizer_x1/2(acc_data)
  [vacc_new_acc] -> packetizer_x1/8(new_acc)
  [vacc_mcnt] -> packetizer_x1/7(mcnt)
  [x_mrst] -> packetizer_x1/1(rst)
  Delay1/1 -> [vacc_dout]
  Delay2/1 -> [vacc_vld]
  Delay3/1 -> [vacc_mcnt]
  Delay446/1 -> packetizer_P/12(delay3)
  Delay447/1 -> packetizer_P/13(power_x0)
  Delay448/1 -> packetizer_P/14(power_y0)
  Delay449/1 -> packetizer_P/15(power_x1)
  Delay45/1 -> packetizer_P/4(acc_len)
  Delay450/1 -> packetizer_P/16(power_y1)
  Delay451/1 -> packetizer_P/17(power2_x0)
  Delay452/1 -> packetizer_P/18(power2_y0)
  Delay453/1 -> packetizer_P/19(power2_x1)
  Delay454/1 -> packetizer_P/20(power2_y1)
  Delay455/1 -> packetizer_P/21(clip_count)
  Delay31/1 -> packetizer_P/2(acc_data)
  Delay43/1 -> packetizer_P/3(acc_valid)
  Delay65/1 -> packetizer_P/22(interpacket_delay)
  Delay66/1 -> packetizer_P/5(use_circular)
  Delay90/1 -> packetizer_P/10(delay1)
  Delay81/1 -> packetizer_P/1(mrst)
  Delay83/1 -> packetizer_P/6(board_id)
  Delay84/1 -> packetizer_P/7(adc_of_count)
  Delay85/1 -> packetizer_P/8(fft_shift)
  Delay89/1 -> packetizer_P/9(delay0)
  Delay97/1 -> packetizer_P/11(delay2)
  Delay4/1 -> Mux/3
  [clr_status] -> Delay5/1
  Delay5/1 -> pfb_fft/9(clear_status)
  Delay7/1 -> FIFO3/3
  Delay9/1 -> FIFO2/3
  Delay10/1 -> FIFO1/3
  Delay11/1 -> FIFO/3
  coarse_delay/1(sync00) -> pfb_fft/3(sync)
  coarse_delay/3(adc0_pol1_out) -> pfb_fft/5(adc0_pol1)
  coarse_delay/2(adc0_pol0_out) -> pfb_fft/4(adc0_pol0)
  coarse_delay/4(adc1_pol0_out) -> pfb_fft/6(adc1_pol0)
  coarse_delay/5(adc1_pol1_out) -> pfb_fft/7(adc1_pol1)
  pfb_fft/10(adc0_pol0_P) -> bus_create/1(in1)
  pfb_fft/11(adc0_pol0_P2) -> bus_create/2(in2)
  pfb_fft/12(adc0_pol1_P) -> bus_create/3(in3)
  pfb_fft/13(adc0_pol1_P2) -> bus_create/4(in4)
  pfb_fft/14(adc1_pol0_P) -> bus_create/5(in5)
  pfb_fft/15(adc1_pol0_P2) -> bus_create/6(in6)
  pfb_fft/16(adc1_pol1_P) -> bus_create/7(in7)
  pfb_fft/17(adc1_pol1_P2) -> bus_create/8(in8)
  bus_create/1(bus_out) -> FIFO/1
  pfb_fft/18(acc_num) -> Terminator20/1
  pfb_fft/19(acc_valid) -> FIFO/2
  pfb_fft/1(sync_out0) -> eq/2(sync)
  eq/1(sync_out_x0) -> [sync_polarimetry_out]
  eq/18(clip_out_x0) -> Logical1/1
  eq/19(clip_out_y0) -> Logical1/2
  eq/20(clip_out_x1) -> Logical1/3
  eq/21(clip_out_y1) -> Logical1/4
  eq/2(quant_even_x0) -> [adc0_pol0_even_q]
  eq/3(quant_odd_x0) -> [adc0_pol0_odd_q]
  eq/4(quant_even_y0) -> [adc0_pol1_even_q]
  eq/5(quant_odd_y0) -> [adc0_pol1_odd_q]
  eq/6(quant_even_x1) -> [adc1_pol0_even_q]
  eq/7(quant_odd_x1) -> [adc1_pol0_odd_q]
  eq/8(quant_even_y1) -> [adc1_pol1_even_q]
  eq/9(quant_odd_y1) -> [adc1_pol1_odd_q]
  eq/10(full_even_x0) -> [adc0_pol0_even]
  eq/12(full_even_y0) -> [adc0_pol1_even]
  eq/13(full_odd_y0) -> [adc0_pol1_odd]
  eq/11(full_odd_x0) -> [adc0_pol0_odd]
  eq/14(full_even_x1) -> [adc1_pol0_even]
  eq/16(full_even_y1) -> [adc1_pol1_even]
  eq/15(full_odd_x1) -> [adc1_pol0_odd]
  eq/17(full_odd_y1) -> [adc1_pol1_odd]
  [adc0_pol1_odd] -> power_cal/5(pol2_f1)
  [adc1_pol0_even] -> power_cal/6(pol3_f0)
  [adc1_pol0_odd] -> power_cal/7(pol3_f1)
  [adc1_pol1_even] -> power_cal/8(pol4_f0)
  [adc1_pol1_odd] -> power_cal/9(pol4_f1)
  [adc0_pol0_even] -> power_cal/2(pol1_f0)
  [adc0_pol0_odd] -> power_cal/3(pol1_f1)
  [adc0_pol1_even] -> power_cal/4(pol2_f0)
  [sync_polarimetry_out] -> power_cal/1(sync_in)
  [ct_tvg] -> Delay30/1
  [adc0_pol0_even_q] -> Delay18/1
  [adc0_pol0_odd_q] -> Delay19/1
  [adc0_pol1_even_q] -> Delay20/1
  [adc0_pol1_odd_q] -> Delay21/1
  [adc1_pol0_even_q] -> Delay22/1
  [adc1_pol1_even_q] -> Delay28/1
  [adc1_pol0_odd_q] -> Delay23/1
  [adc1_pol1_odd_q] -> Delay29/1
  [sync_polarimetry_out] -> Delay17/1
  [acc_start_skip] -> Delay32/1
  [tvg_en] -> Delay34/1
  [acc_len] -> Delay39/1
  [mrst0] -> Delay38/1
  [board_id] -> Delay37/1
  [x_mcnt1] -> Logical3/2
  [x_mcnt0] -> Logical3/1
  [x_dv1] -> Logical2/2
  [x_dv0] -> Logical2/1
  [x_d1] -> Logical4/2
  [x_d0] -> Logical4/1
  [x_sync0] -> Delay6/1
  Logical4/1 -> xeng_hdl_uint/2(ant)
  Logical2/1 -> Delay70/1, xeng_hdl_uint/3(window_valid)
  Logical3/1 -> xeng_hdl_uint/4(mcnt_in)
  xeng_hdl_uint/1(sync_out) -> [all_x_sync]
  xeng_hdl_uint/2(acc) -> [all_x_dout]
  xeng_hdl_uint/3(valid) -> Delay56/1, [all_x_vld]
  xeng_hdl_uint/4(mcnt_out) -> [all_x_mcnt]
  power_cal/2(pol1_f0_pow) -> vector_acc/4(power_in0)
  power_cal/3(pol1_f1_pow) -> vector_acc/5(power_in1)
  power_cal/4(pol2_f0_pow) -> vector_acc/6(power_in2)
  power_cal/5(pol2_f1_pow) -> vector_acc/7(power_in3)
  power_cal/6(pol3_f0_pow) -> vector_acc/8(power_in4)
  power_cal/7(pol3_f1_pow) -> vector_acc/9(power_in5)
  power_cal/8(pol4_f0_pow) -> vector_acc/10(power_in6)
  power_cal/9(pol4_f1_pow) -> vector_acc/11(power_in7)
  power_cal/10(pol1_f0_pow_sq) -> vector_acc/12(sq_power_in0)
  power_cal/11(pol1_f1_pow_sq) -> vector_acc/13(sq_power_in1)
  power_cal/12(pol2_f0_pow_sq) -> vector_acc/14(sq_power_in2)
  power_cal/13(pol2_f1_pow_sq) -> vector_acc/15(sq_power_in3)
  power_cal/14(pol3_f0_pow_sq) -> vector_acc/16(sq_power_in4)
  power_cal/15(pol3_f1_pow_sq) -> vector_acc/17(sq_power_in5)
  power_cal/16(pol4_f0_pow_sq) -> vector_acc/18(sq_power_in6)
  power_cal/17(pol4_f1_pow_sq) -> vector_acc/19(sq_power_in7)
  Constant9/1 -> eq/1(freq_band)
  pfb_fft/2(x0_out0) -> eq/3(x0_even)
  pfb_fft/3(x0_out1) -> eq/4(x0_odd)
  pfb_fft/4(y0_out0) -> eq/5(y0_even)
  pfb_fft/5(y0_out1) -> eq/6(y0_odd)
  pfb_fft/6(x1_out0) -> eq/7(x1_even1)
  pfb_fft/7(x1_out1) -> eq/8(x1_odd1)
  pfb_fft/8(y1_out0) -> eq/9(y1_even1)
  pfb_fft/9(y1_out1) -> eq/10(y1_odd1)
  Delay12/1 -> Delay14/1
  Delay14/1 -> pulse generator1/1(sync)
  Delay15/1 -> FIFO1/1
  Subsystem/6(Out6) -> [mrst5]
  Subsystem/7(Out7) -> [mrst6]
  Subsystem/2(Out2) -> [mrst1]
  Subsystem/8(Out8) -> [mrst7]
  Subsystem/1(Out1) -> [mrst0]
  Subsystem/5(Out5) -> [mrst4]
  Subsystem/3(Out3) -> [mrst2]
  Subsystem/4(Out4) -> [mrst3]
  Constant10/1 -> Rx_Tx_FX0/7
  Constant12/1 -> Rx_Tx_FX0/8
  Constant13/1 -> Rx_Tx_FX1/7
  Constant14/1 -> Rx_Tx_FX1/8
  Delay16/1 -> [delay_val]
  Delay17/1 -> f_x/1(sync)
  Delay18/1 -> f_x/2(ant0_pol0_even)
  Delay19/1 -> f_x/3(ant0_pol0_odd)
  Delay20/1 -> f_x/4(ant0_pol1_even)
  Delay21/1 -> f_x/5(ant0_pol1_odd)
  Delay23/1 -> f_x/7(ant1_pol0_odd)
  Delay28/1 -> f_x/8(ant1_pol1_even)
  Delay22/1 -> f_x/6(ant1_pol0_even)
  Delay38/1 -> f_x/13(mrst)
  Delay29/1 -> f_x/9(ant1_pol1_odd)
  Delay39/1 -> f_x/14(acc_len)
  Delay37/1 -> f_x/12(board_id)
  Delay30/1 -> f_x/10(ct_tvg_in)
  Delay34/1 -> f_x/11(tvg_en_in)
  Delay32/1 -> f_x/15(acc_skip)
  Delay40/1 -> [adc_calibration_data]
  Delay41/1 -> [clip_count]
  [adc1_pol1_odd_q] -> Concat15/2
  [adc1_pol1_odd] -> Concat15/1
  [adc0_pol0_even_q] -> Concat9/2
  [adc0_pol0_even] -> Concat9/1
  [adc0_pol0_odd] -> Concat7/1
  [adc0_pol0_odd_q] -> Concat7/2
  [adc0_pol1_even_q] -> Concat6/2
  [adc0_pol1_even] -> Concat6/1
  [adc0_pol1_odd_q] -> Concat5/2
  [adc0_pol1_odd] -> Concat5/1
  [adc1_pol0_even_q] -> Concat4/2
  [adc1_pol0_even] -> Concat4/1
  [adc1_pol0_odd_q] -> Concat3/2
  [adc1_pol0_odd] -> Concat3/1
  [adc1_pol1_even] -> Concat2/1
  [adc1_pol1_even_q] -> Concat2/2
  Concat9/1 -> Delay42/1
  Concat7/1 -> Delay47/1
  Concat6/1 -> Delay49/1
  Concat5/1 -> Delay50/1
  Concat4/1 -> Delay51/1
  Concat3/1 -> Delay52/1
  Concat2/1 -> Delay53/1
  BitBasher1/1 -> pol_snap/1(din)
  Delay335/1 -> Mux11/1
  Delay44/1 -> Delay13/1, clip_count/1
  Delay46/1 -> clip_count/2
  Delay13/1 -> FIFO1/2
  Delay42/1 -> Mux11/2
  Delay47/1 -> Mux11/3
  Delay49/1 -> Mux11/4
  Delay50/1 -> Mux11/5
  Delay51/1 -> Mux11/6
  Delay52/1 -> Mux11/7
  Delay53/1 -> Mux11/8
  Delay55/1 -> Mux11/9
  Rx_Tx_FX0/12 -> Terminator71/1
  Constant11/1 -> ip1/3(we)
  Constant15/1 -> ip1/2(data_in)
  Constant16/1 -> ip0/3(we)
  Constant19/1 -> ip0/2(data_in)
  Convert5/1 -> ip0/1(addr)
  Slice14/1 -> rx_packet_count_fx0/1(out_reg)
  [gbe_rxvld1] -> Counter1/1
  Counter1/1 -> Slice15/1
  Slice15/1 -> rx_packet_count_fx1/1(out_reg)
  Delay57/1 -> tx_p_overflow/1(out_reg)
  Delay59/1 -> tx_x_overflow/1(out_reg)
  packet_buffer1/1(sync) -> masker2/1(sync)
  masker2/2(dout) -> [x_d1]
  masker2/3(vld_out) -> [x_dv1]
  masker2/1(sync_out) -> [x_sync1]
  masker2/4(mcnt_out) -> [x_mcnt1]
  packet_buffer0/1(sync) -> masker1/1(sync)
  packet_buffer0/2(d0) -> masker1/2(din)
  packet_buffer0/3(dv0) -> masker1/3(vld)
  packet_buffer0/4(mcnt_out0) -> masker1/4(mcnt)
  masker1/4(mcnt_out) -> [x_mcnt0]
  masker1/3(vld_out) -> [x_dv0]
  masker1/2(dout) -> [x_d0]
  masker1/1(sync_out) -> [x_sync0]
  Delay6/1 -> Delay69/1, xeng_hdl_uint/1(sync_in)
  packet_buffer0/7(rd_valid_out1) -> [rd_valid1]
  packet_buffer1/2(d0) -> masker2/2(din)
  packet_buffer1/3(dv0) -> masker2/3(vld)
  packet_buffer1/4(mcnt_out0) -> masker2/4(mcnt)
  Slice16/1 -> x_out_count/1(out_reg)
  Delay56/1 -> Counter50/1
  Slice17/1 -> x_dv_count0/1(out_reg)
  Delay58/1 -> Counter40/1
  Counter2/1 -> Slice18/1
  Slice18/1 -> x_dv_count1/1(out_reg)
  Delay60/1 -> Counter2/1
  [x_dv0] -> Delay58/1
  [x_dv1] -> Delay60/1
  Delay61/1 -> Logical14/1
  Delay64/1 -> Logical14/2
  Delay67/1 -> Logical16/1
  Delay68/1 -> Logical16/2
  Delay70/1 -> Counter3/2
  Delay69/1 -> Register/2, Counter3/1
  Counter3/1 -> Register/1
  Register/1 -> x_in_sync_count/1(out_reg)
